simulink model "xyz_missile_model"  (R2023a)
settings: Solver=VariableStepAuto  StartTime=0.0  StopTime=2.25  RelTol=1e-3
values from neighbouring files (symbols this model uses):
  g = 9.8    [Inital.m]
  Ixx = 0.04    [Inital.m]
  Iyy = 0.4    [Inital.m]
  Izz = 0.4    [Inital.m]
  M = 5    [Inital.m]
  P = 50    [Inital.m]
  pitch0 = 0    [Inital.m]
  psi0 = 3.14/7    (= 0.448571428571)    [Inital.m]
  roll0 = 0    [Inital.m]
  V0 = 30    [Inital.m]
  wx0 = 0    [Inital.m]
  wy0 = 0    [Inital.m]
  wz0 = 0    [Inital.m]
  x0 = 0    [Inital.m]
  Xtar = 100    [Inital.m]
  y0 = 30    [Inital.m]
  yaw0 = 3.14/7    (= 0.448571428571)    [Inital.m]
  Ytar = 0    [Inital.m]
  z0 = 0    [Inital.m]
  zeta0 = 0    [Inital.m]
  Ztar = 0    [Inital.m]
libraries: slpidlib x1
settings Model: Creator=Lenovo  LastModifiedBy=Lenovo

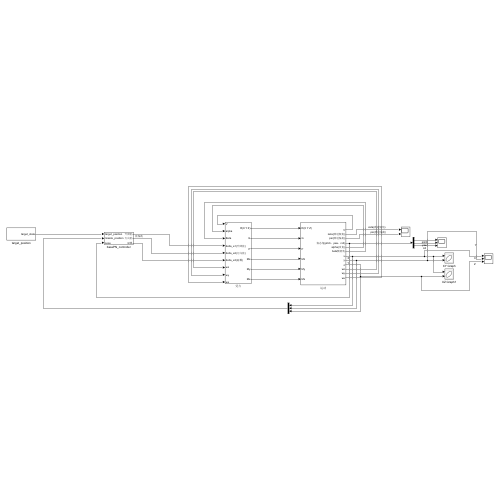
[thumbnail: Simulink's stored preview of the top-level diagram]
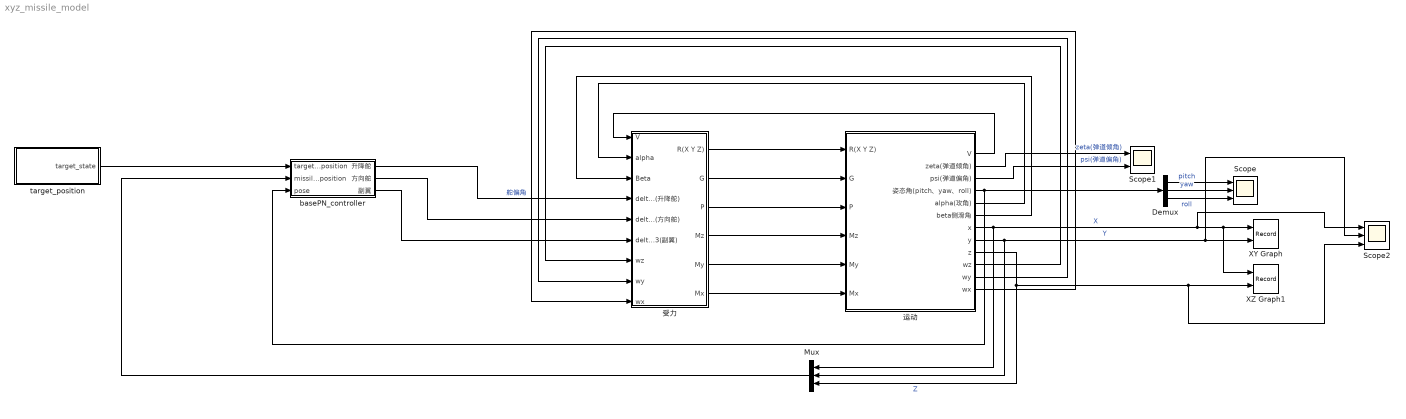
== system xyz_missile_model ==
  Demux : Demux  Outputs=3
  Mux : Mux  Inputs=3
  Scope : Scope  NumInputPorts=3
  Scope1 : Scope  NumInputPorts=2
  Scope2 : Scope  NumInputPorts=3
  XY Graph : Record  FileSettingsInternal="{\"entries\":[{\"content\":{\"excelSettings\":{\"content\":{},\"type\":\"Streamout.ExcelSettings\"}},\"type\":\"Streamout.FileSettingStorage\",\"uuid\":\"50788435-4e7f-4ae6-926e-53e50006c5cf\"}],\"packageUris\":[\"http://schema.mathworks.com/mf0/streamout_blocks/R2020a\"],\"version\":\"1.0\"}"  Layout=[1 1]  SignalsInternal="{\"entries\":[{\"content\":{\"signals\":[{\"content\":{\"blockPath\":[\"xyz_missile_model/XY Graph\"],\"dimensions\":[1],\"domain\":\"xyz_missile_model/XY Graph\",\"lineColor\":\"#a2142f\",\"plots\":[1],\"port\":1,\"signalID\":345,\"signalName\":\"X\"},\"type\":\"RecordBlkView.Signal\",\"uuid\":\"dcb0110f-8eb4-40a9-b5a5-296dc31861ea\"},{\"content\":{\"blockPath\":[\"xyz_missile_model/XY Graph\"],\"dimensions\":[1],\"domain\":\"xyz_missile_model/XY Graph\",\"lineColor\":\"#139fff\",\"plots\":[1],\"port\":2,\"signalID\":348,\"signalName\":\"Y\"},\"type\":\"RecordBlkView.Signal\",\"uuid\":\"65febf6e-97d6-41fd-ba24-90fb87080eb0\"}]},\"type\":\"RecordBlkView.InputSignals\",\"uuid\":\"91050016-8fd4-4e92-80d9-7d87fcb20894\"}],\"packageUris\":[\"http://schema.mathworks.com/mf0/streamout_blocks/R2020a\"],\"version\":\"1.0\"}"  VisualizationBindings="{\"xyplotplugin\":{\"info\":[{\"series\":[{\"bindingParametersList\":[{\"parameter\":\"X-Axis\",\"signalID\":345,\"signalName\":\"X\"},{\"parameter\":\"Y-Axis\",\"signalID\":348,\"signalName\":\"Y\"}],\"seriesID\":40790}],\"subplotID\":1}]}}"  CompatibilityTag=XY  st=-1
  XZ Graph1 : Record  FileSettingsInternal="{\"entries\":[{\"content\":{\"excelSettings\":{\"content\":{},\"type\":\"Streamout.ExcelSettings\"}},\"type\":\"Streamout.FileSettingStorage\",\"uuid\":\"9845f7a1-d993-447e-b346-9c4ab6f3d264\"}],\"packageUris\":[\"http://schema.mathworks.com/mf0/streamout_blocks/R2020a\"],\"version\":\"1.0\"}"  Layout=[1 1]  SignalsInternal="{\"entries\":[{\"content\":{\"signals\":[{\"content\":{\"blockPath\":[\"xyz_missile_model/XZ Graph1\"],\"dimensions\":[1],\"domain\":\"xyz_missile_model/XZ Graph1\",\"lineColor\":\"#a2142f\",\"plots\":[1],\"port\":1,\"signalID\":337,\"signalName\":\"X\"},\"type\":\"RecordBlkView.Signal\",\"uuid\":\"be30e74f-d4c8-4c61-9f2d-d22df2742b39\"},{\"content\":{\"blockPath\":[\"xyz_missile_model/XZ Graph1\"],\"dimensions\":[1],\"domain\":\"xyz_missile_model/XZ Graph1\",\"lineColor\":\"#139fff\",\"plots\":[1],\"port\":2,\"signalID\":340,\"signalName\":\"Z\"},\"type\":\"RecordBlkView.Signal\",\"uuid\":\"4855943b-fddb-41b8-b941-40637d8bbf2a\"}]},\"type\":\"RecordBlkView.InputSignals\",\"uuid\":\"ad51cbb5-b85d-409f-89ef-9a2bae2ee352\"}],\"packageUris\":[\"http://schema.mathworks.com/mf0/streamout_blocks/R2020a\"],\"version\":\"1.0\"}"  VisualizationBindings="{\"xyplotplugin\":{\"info\":[{\"series\":[{\"bindingParametersList\":[{\"parameter\":\"X-Axis\",\"signalID\":337,\"signalName\":\"X\"},{\"parameter\":\"Y-Axis\",\"signalID\":340,\"signalName\":\"Z\"}],\"seriesID\":33451}],\"subplotID\":1}]}}"  CompatibilityTag=XY  st=-1
  basePN_controller : Subsystem
  target_position : Subsystem
  受力 : Subsystem
  运动 : Subsystem
  wires:
  受力/1(R(X Y Z)) -> 运动/1(R(X Y Z))
  受力/2(G) -> 运动/2(G)
  受力/3(P) -> 运动/3(P)
  受力/4(Mz) -> 运动/4(Mz)
  受力/5(My) -> 运动/5(My)
  受力/6(Mx) -> 运动/6(Mx)
  运动/5(alpha(攻角)) -> 受力/2(alpha)
  运动/6(beta侧滑角) -> 受力/3(Beta)
  运动/1(V) -> 受力/1(V)
  运动/10(wz) -> 受力/7(wz)
  运动/11(wy) -> 受力/8(wy)
  运动/12(wx) -> 受力/9(wx)
  basePN_controller/2(方向舵) -> 受力/5(delta_e2(方向舵))
  basePN_controller/3(副翼) -> 受力/6(delta_e3(副翼))
  target_position/1(target_state) -> basePN_controller/1(target_position)
  运动/7(x) -> Mux/1, Scope2/1, XZ Graph1/1, XY Graph/1  "X"
  运动/8(y) -> Mux/2, Scope2/2, XY Graph/2  "Y"
  Mux/1 -> basePN_controller/2(missile_position)
  basePN_controller/1(升降舵) -> 受力/4(delta_e1(升降舵))  "舵偏角"
  运动/9(z) -> Scope2/3, XZ Graph1/2, Mux/3  "Z"
  运动/2(zeta(弹道倾角)) -> Scope1/1  "zeta(弹道倾角)"
  运动/3(psi(弹道偏角)) -> Scope1/2  "psi(弹道偏角)"
  运动/4(姿态角(pitch、yaw、roll)) -> Demux/1, basePN_controller/3(pose)
  Demux/1 -> Scope/1  "pitch"
  Demux/2 -> Scope/2  "yaw"
  Demux/3 -> Scope/3  "roll"

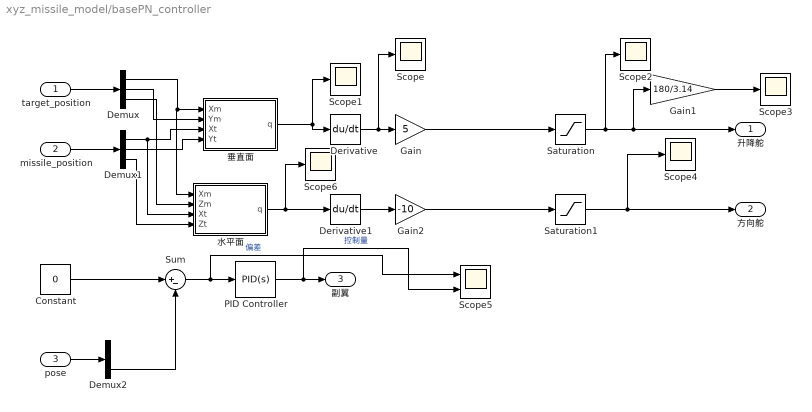
== system xyz_missile_model/basePN_controller ==
  target_position : Inport
  missile_position : Inport  Port=2
  pose : Inport  Port=3
  Constant : Constant  Value=0
  Demux : Demux  Outputs=3
  Demux1 : Demux  Outputs=3
  Demux2 : Demux  Outputs=3
  Derivative : Derivative
  Derivative1 : Derivative
  Gain : Gain  Gain=5
  Gain1 : Gain  Gain=180/3.14
  Gain2 : Gain  Gain=-10
  PID Controller : slpidlib/PID Controller  Controller=PID  Form=Parallel  TimeDomain=Continuous-time  UseExternalTs=off  SampleTime=-1  IntegratorMethod=Forward Euler  FilterMethod=Forward Euler  ControllerParametersSource=internal  P=1.5  I=0  UseKiTs=off  D=2  N=100  UseFilter=on  TunerSelectOption=Transfer Function Based (PID Tuner App)  InitialConditionSource=internal  InitialConditionForIntegrator=0  InitialConditionForFilter=0  DifferentiatorICPrevScaledInput=0  ExternalReset=none  TrackingMode=off  Kt=1  LimitOutput=on  SatLimitsSource=internal  UpperSaturationLimit=3.14/4  LowerSaturationLimit=3.14/-4  LinearizeAsGain=on  AntiWindupMode=none  Kb=1  LimitIntegrator=on  UpperIntegratorSaturationLimit=3.14/6  LowerIntegratorSaturationLimit=-3.14/6  POutMin=[]  POutMax=[]  IOutMin=[]  IOutMax=[]  DOutMin=[]  DOutMax=[]  NOutMin=[]  NOutMax=[]  SumOutMin=[]  SumOutMax=[]  SaturationOutMin=[]  SaturationOutMax=[]  PParamMin=[]  PParamMax=[]  IParamMin=[]  IParamMax=[]  DParamMin=[]  DParamMax=[]  NParamMin=[]  NParamMax=[]  KbParamMin=[]  KbParamMax=[]  KtParamMin=[]  KtParamMax=[]  KbOutMin=[]  KbOutMax=[]  KtOutMin=[]  KtOutMax=[]  IntegratorOutMin=[]  IntegratorOutMax=[]  FilterOutMin=[]  FilterOutMax=[]  SumI1OutMin=[]  SumI1OutMax=[]  SumI2OutMin=[]  SumI2OutMax=[]  SumI3OutMin=[]  SumI3OutMax=[]  SumI4OutMin=[]  SumI4OutMax=[]  SumDOutMin=[]  SumDOutMax=[]  DifferentiatorOutMin=[]  DifferentiatorOutMax=[]  FilterDiffOutCoefMin=[]  FilterDiffOutCoefMax=[]  ReciprocalOutMin=[]  ReciprocalOutMax=[]  SumDenOutMin=[]  SumDenOutMax=[]  SumNumOutMin=[]  SumNumOutMax=[]  DivideOutMin=[]  DivideOutMax=[]  UdiffTsProdOutMin=[]  UdiffTsProdOutMax=[]  NTsProdOutMin=[]  NTsProdOutMax=[]  UintegralTsProdOutMin=[]  UintegralTsProdOutMax=[]  UngainTsProdOutMin=[]  UngainTsProdOutMax=[]  ClampingZeroOutDataTypeStr=Inherit: Inherit via back propagation  ClampingZeroOutMin=[]  ClampingZeroOutMax=[]  FilterDenConstantOutDataTypeStr=Inherit: Inherit via back propagation  FilterDenConstantOutMin=[]  FilterDenConstantOutMax=[]  PCopyOutDataTypeStr=Inherit: Inherit via back propagation  PCopyOutMin=[]  PCopyOutMax=[]  NCopyOutDataTypeStr=Inherit: Inherit via back propagation  NCopyOutMin=[]  NCopyOutMax=[]  IntegratorContinuousStateAttributes=''  IntegratorStateMustResolveToSignalObject=off  IntegratorRTWStateStorageClass=Auto  FilterContinuousStateAttributes=''  FilterStateMustResolveToSignalObject=off  FilterRTWStateStorageClass=Auto  ParallelPVariant=InternalParameters  IdealPVariant=Disabled  IVariant=InternalParameters  DVariant=InternalParameters  IntegratorVariant=Continuous  SatVariant=Enabled  AWVariant=Passthrough  PCopyVariant=Disabled  TRVariant=Disabled  FdbkBlocksVariant=Forward  IdealPFdbkVariant=Disabled  SatFdbkVariant=Disabled  DerivativeFilterVariant=ContFilter  NVariant=InternalParameters  NCopyVariant=Disabled  FilterICVariant=InternalICsFilter  IntegratorICVariant=InternalICs  ExternalResetVariant=Disabled  TRSumVariant=Passthrough  SumFdbkVariant=Disabled  SumVariant=Sum_PID  TsampFilterVariant=InternalTs  TsampNgainVariant=Passthrough  TsampIntegralVariant=Disabled_SignalSpec  ExternalSaturationOutDataTypeStr=Inherit: Same as second input
  Saturation : Saturate  UpperLimit=3.14/3  LowerLimit=-3.14/3
  Saturation1 : Saturate  UpperLimit=3.14/4  LowerLimit=-3.14/4
  Scope{,1..4,6} (6 alike) : Scope
  Scope5 : Scope  NumInputPorts=2
  Sum : Sum  Inputs=|+-
  垂直面 : MATLAB Function  TreatAsAtomicUnit=on
  水平面 : MATLAB Function  TreatAsAtomicUnit=on
  升降舵 : Outport
  方向舵 : Outport  Port=2
  副翼 : Outport  Port=3
  wires:
  target_position/1 -> Demux/1
  missile_position/1 -> Demux1/1
  Demux1/1 -> 水平面/3(Xt), 垂直面/3(Xt)
  Demux1/2 -> 垂直面/4(Yt)
  Demux/1 -> 垂直面/1(Xm), 水平面/1(Xm)
  Demux/2 -> 垂直面/2(Ym)
  垂直面/1(q) -> Derivative/1, Scope1/1
  Derivative/1 -> Scope/1, Gain/1
  Gain/1 -> Saturation/1
  Gain1/1 -> Scope3/1
  Saturation/1 -> Scope2/1, 升降舵/1, Gain1/1
  Demux/3 -> 水平面/2(Zm)
  Demux1/3 -> 水平面/4(Zt)
  水平面/1(q) -> Scope6/1, Derivative1/1
  Derivative1/1 -> Gain2/1
  Gain2/1 -> Saturation1/1
  Saturation1/1 -> Scope4/1, 方向舵/1
  pose/1 -> Demux2/1
  Demux2/3 -> Sum/2
  Constant/1 -> Sum/1
  Sum/1 -> Scope5/1, PID Controller/1  "偏差"
  PID Controller/1 -> Scope5/2, 副翼/1  "控制量"

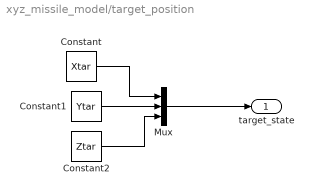
== system xyz_missile_model/target_position ==
  Constant : Constant  Value=Xtar
  Constant1 : Constant  Value=Ytar
  Constant2 : Constant  Value=Ztar
  Mux : Mux  Inputs=3
  target_state : Outport
  wires:
  Constant/1 -> Mux/1
  Constant1/1 -> Mux/2
  Mux/1 -> target_state/1
  Constant2/1 -> Mux/3

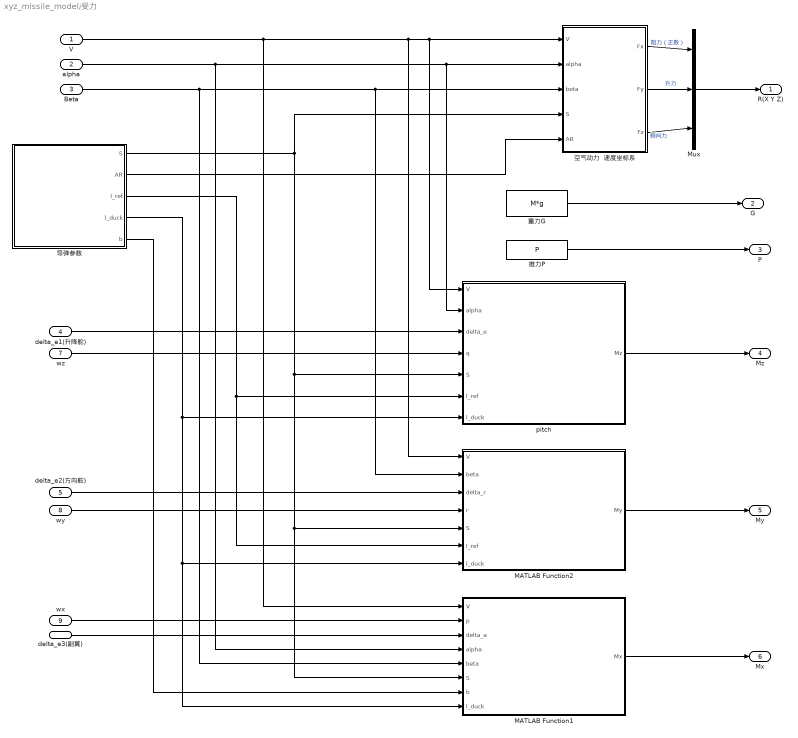
== system xyz_missile_model/受力 ==
  V : Inport
  alpha : Inport  Port=2
  Beta : Inport  Port=3
  delta_e1(升降舵) : Inport  Port=4
  delta_e2(方向舵) : Inport  Port=5
  delta_e3(副翼) : Inport  Port=6
  wz : Inport  Port=7
  wy : Inport  Port=8
  wx : Inport  Port=9
  MATLAB Function1 : MATLAB Function  TreatAsAtomicUnit=on
  MATLAB Function2 : MATLAB Function  TreatAsAtomicUnit=on
  Mux : Mux  Inputs=3
  pitch : MATLAB Function  TreatAsAtomicUnit=on
  导弹参数 : Subsystem
  推力P : Constant  Value=P
  空气动力  速度坐标系 : MATLAB Function  TreatAsAtomicUnit=on
  重力G : Constant  Value=M*g
  R(X Y Z) : Outport
  G : Outport  Port=2
  P : Outport  Port=3
  Mz : Outport  Port=4
  My : Outport  Port=5
  Mx : Outport  Port=6
  wires:
  空气动力  速度坐标系/3(Fz) -> Mux/3  "侧向力"
  空气动力  速度坐标系/2(Fy) -> Mux/2  "升力"
  空气动力  速度坐标系/1(Fx) -> Mux/1  "阻力（正数）"
  Beta/1 -> MATLAB Function1/5(beta), MATLAB Function2/2(beta), 空气动力  速度坐标系/3(beta)
  Mux/1 -> R(X Y Z)/1
  重力G/1 -> G/1
  推力P/1 -> P/1
  V/1 -> MATLAB Function1/1(V), MATLAB Function2/1(V), 空气动力  速度坐标系/1(V), pitch/1(V)
  alpha/1 -> MATLAB Function1/4(alpha), 空气动力  速度坐标系/2(alpha), pitch/2(alpha)
  pitch/1(Mz) -> Mz/1
  wz/1 -> pitch/4(q)
  delta_e1(升降舵)/1 -> pitch/3(delta_e)
  导弹参数/1(S) -> MATLAB Function2/5(S), MATLAB Function1/6(S), pitch/5(S), 空气动力  速度坐标系/4(S)
  导弹参数/2(AR) -> 空气动力  速度坐标系/5(AR)
  导弹参数/3(l_ref) -> pitch/6(l_ref), MATLAB Function2/6(l_ref)
  导弹参数/4(l_duck) -> MATLAB Function1/8(l_duck), MATLAB Function2/7(l_duck), pitch/7(l_duck)
  delta_e3(副翼)/1 -> MATLAB Function1/3(delta_a)
  delta_e2(方向舵)/1 -> MATLAB Function2/3(delta_r)
  wy/1 -> MATLAB Function2/4(r)
  wx/1 -> MATLAB Function1/2(p)
  导弹参数/5(b) -> MATLAB Function1/7(b)
  MATLAB Function2/1(My) -> My/1
  MATLAB Function1/1(Mx) -> Mx/1

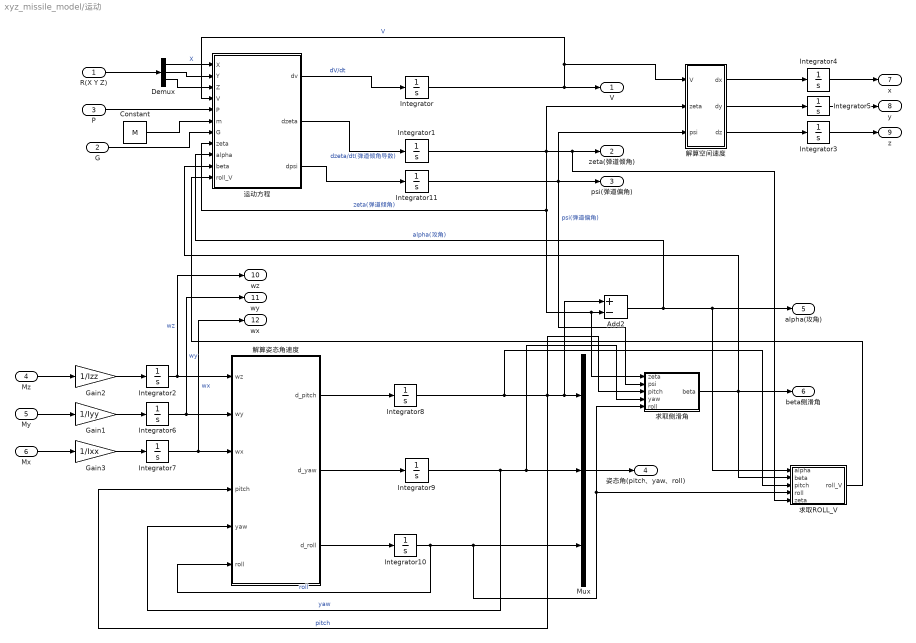
== system xyz_missile_model/运动 ==
  R(X Y Z) : Inport
  G : Inport  Port=2
  P : Inport  Port=3
  Mz : Inport  Port=4
  My : Inport  Port=5
  Mx : Inport  Port=6
  Add2 : Sum  Inputs=+-
  Constant : Constant  Value=M
  Demux : Demux  Outputs=3
  Gain1 : Gain  Gain=1/Iyy
  Gain2 : Gain  Gain=1/Izz
  Gain3 : Gain  Gain=1/Ixx
  Integrator : Integrator  InitialCondition=V0
  Integrator1 : Integrator  InitialCondition=zeta0
  Integrator10 : Integrator  InitialCondition=roll0
  Integrator11 : Integrator  InitialCondition=psi0
  Integrator2 : Integrator  InitialCondition=wz0
  Integrator3 : Integrator  InitialCondition=z0
  Integrator4 : Integrator  InitialCondition=x0
  Integrator5 : Integrator  InitialCondition=y0
  Integrator6 : Integrator  InitialCondition=wy0
  Integrator7 : Integrator  InitialCondition=wx0
  Integrator8 : Integrator  InitialCondition=pitch0
  Integrator9 : Integrator  InitialCondition=yaw0
  Mux : Mux  Inputs=3
  求取ROLL_V : MATLAB Function  TreatAsAtomicUnit=on
  求取侧滑角 : MATLAB Function  TreatAsAtomicUnit=on
  解算姿态角速度 : MATLAB Function  TreatAsAtomicUnit=on
  解算空间速度 : MATLAB Function  TreatAsAtomicUnit=on
  运动方程 : MATLAB Function  TreatAsAtomicUnit=on
  V : Outport
  zeta(弹道倾角) : Outport  Port=2
  psi(弹道偏角) : Outport  Port=3
  姿态角(pitch、yaw、roll) : Outport  Port=4
  alpha(攻角) : Outport  Port=5
  beta侧滑角 : Outport  Port=6
  x : Outport  Port=7
  y : Outport  Port=8
  z : Outport  Port=9
  wz : Outport  Port=10
  wy : Outport  Port=11
  wx : Outport  Port=12
  wires:
  R(X Y Z)/1 -> Demux/1
  P/1 -> 运动方程/5(P)
  运动方程/1(dv) -> Integrator/1  "dV/dt"
  运动方程/2(dzeta) -> Integrator1/1  "dzeta/dt(弹道倾角导数)"
  Integrator1/1 -> 求取侧滑角/1(zeta), Add2/2, 运动方程/8(zeta), 解算空间速度/2(zeta), 求取ROLL_V/5(zeta), zeta(弹道倾角)/1  "zeta(弹道倾角)"
  Mz/1 -> Gain2/1
  Gain2/1 -> Integrator2/1
  Add2/1 -> 运动方程/9(alpha), 求取ROLL_V/1(alpha), alpha(攻角)/1  "alpha(攻角)"
  Demux/1 -> 运动方程/1(X)  "X"
  Demux/2 -> 运动方程/2(Y)
  G/1 -> 运动方程/7(G)
  Constant/1 -> 运动方程/6(m)
  Integrator4/1 -> x/1
  Integrator5/1 -> y/1
  Integrator/1 -> 解算空间速度/1(V), 运动方程/4(V), V/1  "V"
  My/1 -> Gain1/1
  Mx/1 -> Gain3/1
  Gain1/1 -> Integrator6/1
  Gain3/1 -> Integrator7/1
  Integrator8/1 -> 求取ROLL_V/3(pitch), 求取侧滑角/3(pitch), Add2/1, Mux/1, 解算姿态角速度/4(pitch)  "pitch"
  Integrator9/1 -> 解算姿态角速度/5(yaw), 求取侧滑角/4(yaw), Mux/2  "yaw"
  Integrator10/1 -> 解算姿态角速度/6(roll), 求取ROLL_V/4(roll), 求取侧滑角/5(roll), Mux/3  "roll"
  Integrator6/1 -> wy/1, 解算姿态角速度/2(wy)  "wy"
  Integrator7/1 -> wx/1, 解算姿态角速度/3(wx)  "wx"
  Integrator2/1 -> wz/1, 解算姿态角速度/1(wz)  "wz"
  解算姿态角速度/1(d_pitch) -> Integrator8/1
  解算姿态角速度/2(d_yaw) -> Integrator9/1
  解算姿态角速度/3(d_roll) -> Integrator10/1
  Mux/1 -> 姿态角(pitch、yaw、roll)/1
  Integrator3/1 -> z/1
  Demux/3 -> 运动方程/3(Z)
  运动方程/3(dpsi) -> Integrator11/1
  Integrator11/1 -> 求取侧滑角/2(psi), 解算空间速度/3(psi), psi(弹道偏角)/1  "psi(弹道偏角)"
  解算空间速度/1(dx) -> Integrator4/1
  解算空间速度/2(dy) -> Integrator5/1
  解算空间速度/3(dz) -> Integrator3/1
  求取侧滑角/1(beta) -> 运动方程/10(beta), 求取ROLL_V/2(beta), beta侧滑角/1
  求取ROLL_V/1(roll_V) -> 运动方程/11(roll_V)

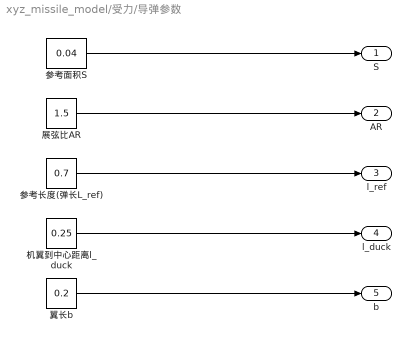
== system xyz_missile_model/受力/导弹参数 ==
  参考长度(弹长L_ref) : Constant  Value=0.7
  参考面积S : Constant  Value=0.04
  展弦比AR : Constant  Value=1.5
  机翼到中心距离l_duck : Constant  Value=0.25
  翼长b : Constant  Value=0.2
  S : Outport
  AR : Outport  Port=2
  l_ref : Outport  Port=3
  l_duck : Outport  Port=4
  b : Outport  Port=5
  wires:
  参考长度(弹长L_ref)/1 -> l_ref/1
  参考面积S/1 -> S/1
  展弦比AR/1 -> AR/1
  翼长b/1 -> b/1
  机翼到中心距离l_duck/1 -> l_duck/1

== matlab function xyz_missile_model/运动/解算空间速度 ==
  data: V input; dx output; zeta input; psi input; dy output; dz output
function [dx,dy,dz]= fcn(V,zeta,psi)

dx=V*cos(zeta);
dy=V*sin(zeta);
dz=-V*cos(zeta)*sin(psi);
end

== matlab function xyz_missile_model/运动/求取侧滑角 ==
  data: zeta input; psi input; beta output; pitch input; yaw input; roll input
function beta = fcn(zeta,psi,pitch,yaw,roll)
t=cos(zeta)*(cos(roll)*sin(yaw-psi)+sin(pitch)*sin(roll)*cos(yaw-psi)-sin(zeta)*cos(pitch)*sin(roll));
beta=asin(t);
end

== matlab function xyz_missile_model/运动/求取ROLL_V ==
  data: alpha input; roll_V output; beta input; pitch input; roll input; zeta input
function roll_V = fcn(alpha,beta,pitch,roll,zeta)
t=( ...
    cos(alpha)*sin(beta)*sin(pitch) ...
    -sin(alpha)*sin(beta)*cos(roll)*cos(pitch) ...
    +cos(beta)*sin(roll)*cos(pitch) ...
    )/cos(zeta);
roll_V=asin(t);
end

== matlab function xyz_missile_model/basePN_controller/垂直面 ==
  data: Xm input; q output; Ym input; Xt input; Yt input
function q = fcn(Xm,Ym,Xt,Yt)
q=atan((Yt-Ym)/(Xt-Xm));
end

== matlab function xyz_missile_model/basePN_controller/水平面 ==
  data: Xm input; q output; Zm input; Xt input; Zt input
function q = fcn(Xm,Zm,Xt,Zt)
q=atan((Zt-Zm)/(Xt-Xm));
end

== matlab function xyz_missile_model/受力/pitch ==
  data: V input; Mz output; alpha input; delta_e input; q input; S input; l_ref input; l_duck input
function Mz = calc_pitch_moment_duck(V, alpha, delta_e, q, S, l_ref, l_duck)
    % 鸭式布局导弹俯仰力矩计算（绕Y轴）
    % 输入参数：
    %   状态参数：
    %   V       - 导弹飞行速度 (m/s)
    %   alpha   - 攻角 (rad)
    %   delta_e - 鸭式升降舵偏角 (rad，正为上偏)
    %   q       - 俯仰角速度 (rad/s)
    %   几何参数（可调整）：
    %   S       - 参考面积 (m²)
    %   l_ref   - 弹体参考长度（弹长）(m)
    %   l_duck  - 鸭翼到重心距离 (m)
    % 输出参数：
    %   Mz      - 俯仰力矩 (N·m)
    
    % 参数有效性检查
    if S <= 0 || l_ref <= 0 || l_duck <= 0
        error('Geometry parameters must be positive values');
    end
    if V < 0
        error('Velocity cannot be negative');
    end
    
    % 气动系数（鸭式布局推荐值）
    c_m_alpha = -0.7;    % 攻角导数 (1/rad)，推荐-0.6~-0.8
    c_m_delta = 0.5;     % 鸭翼舵偏导数 (1/rad)，推荐0.4~0.6（正值：上偏产生抬头力矩）
    c_m_q = -2.3;        % 俯仰角速度阻尼 (1/rad)，推荐-2.0~-2.5
    c_m_duck_couple = 0.2; % 鸭翼-攻角耦合项 (1/rad²)
    
    % 空气密度（50m高度）
    rho = 1.225;
    
    % 动态压
    dynamic_pressure = 0.5 * rho * V^2;
    
    % 无量纲俯仰角速度
    if V<1
        q_hat=0;
    else
        q_hat=(q * l_ref) / (2 * V);
    end
    
    % 俯仰力矩系数（鸭式布局专用）
    Cm = c_m_alpha * alpha ...
        + c_m_delta * delta_e ...  % 鸭翼舵偏产生同向力矩（与尾翼相反）
        + c_m_q * q_hat ...
        + c_m_duck_couple * alpha * delta_e;  % 鸭翼-攻角耦合效应
    
    % 计算最终俯仰力矩
    Mz = dynamic_pressure * S * l_ref * Cm;
end

== matlab function xyz_missile_model/受力/空气动力  速度坐标系 ==
  data: V input; Fx output; alpha input; beta input; S input; AR input; Fy output; Fz output
function [Fx, Fy, Fz] = missile_forces(V, alpha, beta, S, AR)
    % 计算速度坐标系下的导弹空气动力
    % 输入参数：
    %   V - 导弹速度大小 (m/s)
    %   alpha - 攻角 (rad)
    %   beta - 侧滑角 (rad)
    %   S - 参考面积 (m²)
    %   AR - 展弦比
    % 输出参数：
    %   Fx - 阻力 (-X方向，与速度方向相反)
    %   Fy - 升力 (Y方向，垂直速度向上)
    %   Fz - 侧向力 (Z方向，垂直速度侧向)
    
    % 1. 空气密度（50m高度近似为海平面值）
    rho = 1.225;  % kg/m³
    
    % 2. 升力计算
    % 升力系数 (小攻角线性模型)
    CL_alpha = 4.0;  % 升力线斜率 (1/rad)
    CL = CL_alpha * alpha;  % 升力系数
    
    % 升力 (Y方向)
    Fy = 0.5 * rho * V^2 * S * CL;
    
    % 3. 阻力计算
    % 零升阻力系数
    CD0 = 0.05;
    
    % 诱导阻力系数
    e = 0.7;  % Oswald效率因子
    CDi = CL^2 / (pi * AR * e);  % 诱导阻力系数
    
    % 总阻力系数
    CD = CD0 + CDi;
    
    % 阻力 (-X方向，与速度方向相反)
    Fx = 0.5 * rho * V^2 * S * CD;  % 
    
    % 4. 侧向力计算
    % 侧力系数 (小侧滑角线性模型)
    CY_beta = -3.5;  % 侧力线斜率 (1/rad)，负号表示侧力方向与侧滑角相反
    CY = CY_beta * beta;  % 侧力系数
    
    % 侧向力 (Z方向)
    Fz = 0.5 * rho * V^2 * S * CY;
end

== matlab function xyz_missile_model/受力/MATLAB Function1 ==
  data: V input; Mx output; p input; delta_a input; alpha input; beta input; S input; b input; l_duck input
function Mx = calc_roll_moment_duck(V, p, delta_a, alpha, beta, S, b, l_duck)
    % 鸭式布局导弹滚动力矩计算（绕X轴）
    % 输入参数：
    %   状态参数：
    %   V       - 导弹飞行速度 (m/s)
    %   p       - 滚转角速度 (rad/s)
    %   delta_a - 鸭式副翼偏角 (rad，正为右鸭翼上偏)
    %   alpha   - 攻角 (rad)
    %   beta    - 侧滑角 (rad)
    %   几何参数（可调整）：
    %   S       - 参考面积 (m²)
    %   b       - 翼展 (m)
    %   l_duck  - 鸭翼到重心距离 (m)
    % 输出参数：
    %   Mx      - 滚动力矩 (N·m)
    
    % 参数有效性检查
    if S <= 0 || b <= 0 || l_duck <= 0
        error('Geometry parameters must be positive values');
    end
    if V < 0
        error('Velocity cannot be negative');
    end
    
    % 气动系数（鸭式布局推荐值）
    c_l_p = -0.6;      % 滚转角速度阻尼 (1/rad)，推荐-0.5~-0.7
    c_l_delta = 0.3;   % 鸭式副翼偏导数 (1/rad)，推荐0.2~0.4（正值：右偏产生右滚转）
    c_l_alpha_beta = 0.7; % 攻角-侧滑角耦合项
    c_l_duck_couple = 0.1; % 鸭翼滚转耦合项
    
    % 空气密度（50m高度）
    rho = 1.225;
    
    % 动态压
    dynamic_pressure = 0.5 * rho * V^2;
    
    % 无量纲滚转角速度
    if V<1
        p_hat=0;
    else
        p_hat=(p * b) / (2 * V);
    end
    
    % 滚动力矩系数（鸭式布局专用）
    Cl = c_l_p * p_hat ...
        + c_l_delta * delta_a ...  % 鸭翼副翼偏角产生同向滚转力矩
        + c_l_alpha_beta * alpha * beta ...
        + c_l_duck_couple * delta_a * (alpha^2 + beta^2);  % 鸭翼非线性耦合
    
    % 计算最终滚动力矩
    Mx = dynamic_pressure * S * b * Cl;
end

== matlab function xyz_missile_model/受力/MATLAB Function2 ==
  data: V input; My output; beta input; delta_r input; r input; S input; l_ref input; l_duck input
function My = calc_yaw_moment_duck(V, beta, delta_r, r, S, l_ref, l_duck)
    % 鸭式布局导弹偏航力矩计算（绕Z轴）
    % 输入参数：
    %   状态参数：
    %   V       - 导弹飞行速度 (m/s)
    %   beta    - 侧滑角 (rad)
    %   delta_r - 鸭式方向舵偏角 (rad，正为右偏)
    %   r       - 偏航角速度 (rad/s)
    %   几何参数（可调整）：
    %   S       - 参考面积 (m²)
    %   l_ref   - 弹体参考长度（弹长）(m)
    %   l_duck  - 鸭翼到重心距离 (m)
    % 输出参数：
    %   My      - 偏航力矩 (N·m)
    
    % 参数有效性检查
    if S <= 0 || l_ref <= 0 || l_duck <= 0
        error('Geometry parameters must be positive values');
    end
    if V < 0
        error('Velocity cannot be negative');
    end
    
    % 气动系数（鸭式布局推荐值，与俯仰对称）
    c_n_beta = -0.7;     % 侧滑角导数 (1/rad)，推荐-0.6~-0.8（与c_m_alpha相同）
    c_n_delta = 0.5;     % 鸭翼方向舵偏导数 (1/rad)，推荐0.4~0.6（与c_m_delta相同）
    c_n_r = -2.3;        % 偏航角速度阻尼 (1/rad)，推荐-2.0~-2.5（与c_m_q相同）
    c_n_duck_couple = 0.2; % 鸭翼-侧滑角耦合项 (1/rad²)
    
    % 空气密度（50m高度）
    rho = 1.225;
    
    % 动态压
    dynamic_pressure = 0.5 * rho * V^2;
    
    % 无量纲偏航角速度
    if V<1
        r_hat=0;
    else
        r_hat= (r * l_ref) / (2 * V);
    end
    
    % 偏航力矩系数（鸭式布局专用）
    Cn = c_n_beta * beta ...
        + c_n_delta * delta_r ...  % 鸭翼方向舵偏产生同向力矩
        + c_n_r * r_hat ...
        + c_n_duck_couple * beta * delta_r;  % 鸭翼-侧滑角耦合效应
    
    % 计算最终偏航力矩
    My = dynamic_pressure * S * l_ref * Cn;
end

== matlab function xyz_missile_model/运动/运动方程 ==
  data: X input; Y input; Z input; V input; P input; m input; G input; zeta input; dv output; alpha input; dzeta output; dpsi output; beta input; roll_V input
function [dv, dzeta,dpsi] = missile_act(X,Y,Z,V,P,m,G,zeta,alpha,beta,roll_V)

    dv=(P*cos(alpha)-X-G*sin(zeta))/m;
    dzeta=(P*sin(alpha)+Y-G*cos(zeta))/(m*V);
    t=(P*sin(alpha)+Y)*sin(roll_V)-(P*cos(alpha)*sin(beta)-Z)*cos(roll_V);
    dpsi=-t/(m*V*cos(zeta));
        
end

== matlab function xyz_missile_model/运动/解算姿态角速度 ==
  data: d_pitch output; wz input; wy input; wx input; d_yaw output; d_roll output; pitch input; yaw input; roll input
function [d_pitch,d_yaw,d_roll]= fcn(wz,wy,wx,pitch,yaw,roll)

d_pitch=wy*sin(roll)+wz*cos(roll);
d_yaw=(wy*cos(roll)-wz*sin(roll))/cos(pitch);
d_roll=wx-tan(pitch)*(wy*cos(roll)-wz*sin(roll));
end
